simulink library "SUB_PLANT_Chassis"  (R2018a)
settings: Solver=VariableStepAuto  StartTime=0.0  StopTime=10.0  RelTol=1e-3
values from neighbouring files (symbols this model uses):
  Cf = 120000    [SUB_PLANT_LateralDynamics_CAL.mat]
  Cr = 240000    [SUB_PLANT_LateralDynamics_CAL.mat]
  GLB_FIXED_STEP_SIZE_CPV = ptc_matlab_lib.PTC_MBDS_Parameter('Value', 0.01,  	'Description', 'Global Fixed Step Size (Fundamental Sample Time)',  	'Unit', 's',  	'CoderInfo.StorageClass', 'Custom',  	'CoderInfo.CustomStorageClass', 'Const')    [GLB_CONST.m]
  heading_0 = 5.2    [SUB_PLANT_LateralDynamics_CAL.mat]
  Iz = 10000    [SUB_PLANT_LateralDynamics_CAL.mat]
  lf = 2.5    [SUB_PLANT_LateralDynamics_CAL.mat]
  lr = 3.5    [SUB_PLANT_LateralDynamics_CAL.mat]
  Vx_0 = 1    [SUB_PLANT_LateralDynamics_CAL.mat]
undefined symbols (not defined in the file or in its folder): DiscIntNeverNeededParam, GLB_TRANS_LOSS_TRQ_GEAR_STEP_MPV, GLB_TRANS_LOSS_TRQ_SPD_STEP_MPV, GLB_TRANS_LOSS_TRQ_TABLE_DATA_MPV, GLB_TRANS_LOSS_TRQ_TRQ_STEP_MPV
libraries: PTC_MBDS_LIB x41, simulink x6
(part 2 of 2)

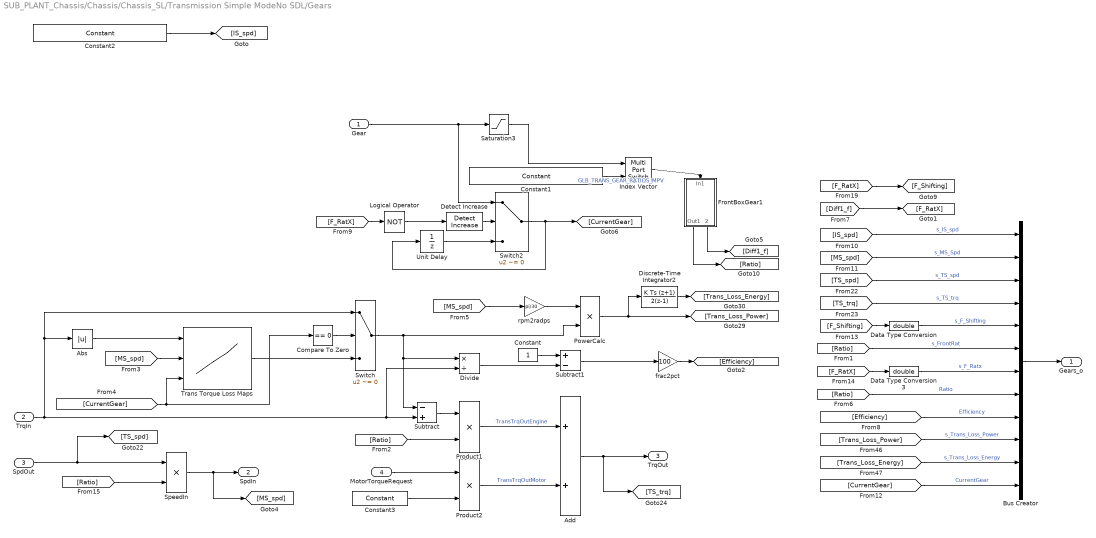
== system SUB_PLANT_Chassis/Chassis/Chassis_SL/Transmission Simple ModeNo SDL/Gears ==
  Gear : Inport
  TrqIn : Inport  Port=2
  SpdOut : Inport  Port=3
  MotorTorqueRequest : Inport  Port=4
  Abs : Abs
  Add : Sum
  Bus Creator : BusCreator  Inputs=12
  Compare To Zero : simulink/Logic and Bit Operations/Compare To Zero  relop===  OutDataTypeStr=boolean
  Constant : Constant
  Constant1 : PTC_MBDS_LIB/Extras/Sources/Constant  Value2=GLB_TRANS_GEAR_RATIOS_MPV  PTC_MBDS_BlockVersion=5.41  PTC_BlockType=PTC_MBDS_Constant
      settings: SourceProductName=PACCAR Technical Center MBDS Library
      settings: AttributesFormatString=|
      | Value: <1 X 12>
      | Unit: '1'
  Constant2 : PTC_MBDS_LIB/Extras/Sources/Constant  Value2=0  PTC_MBDS_BlockVersion=5.41  PTC_BlockType=PTC_MBDS_Constant
      settings: SourceProductName=PACCAR Technical Center MBDS Library
  Constant3 : PTC_MBDS_LIB/Extras/Sources/Constant  Value2=1  PTC_MBDS_BlockVersion=5.41  PTC_BlockType=PTC_MBDS_Constant
      settings: SourceProductName=PACCAR Technical Center MBDS Library
  Data Type Conversion : DataTypeConversion  OutDataTypeStr=double
  Data Type Conversion3 : DataTypeConversion  OutDataTypeStr=double
  Detect Increase : simulink/Logic and Bit Operations/Detect Increase  vinit=0.0  OutDataTypeStr=boolean
  Discrete-Time Integrator2 : DiscreteIntegrator  IntegratorMethod=Integration: Trapezoidal  SampleTime=GLB_FIXED_STEP_SIZE_CPV  ICPrevOutput=DiscIntNeverNeededParam  ICPrevScaledInput=DiscIntNeverNeededParam
  Divide : Product  Inputs=*/
  FrontBoxGear1 : Subsystem
  Index Vector : MultiPortSwitch  Inputs=1
  Logical Operator : Logic  Operator=NOT  AllPortsSameDT=off  OutDataTypeStr=boolean
  PowerCalc : Product
  Product1 : Product
  Product2 : Product
  Saturation3 : Saturate  UpperLimit=inf  LowerLimit=1
  SpeedIn : Product
  Subtract : Sum  Inputs=-+
  Subtract1 : Sum  Inputs=+-
  Switch : Switch  Criteria=u2 ~= 0
  Switch2 : Switch  Criteria=u2 ~= 0
  Trans Torque Loss Maps : Lookup_n-D  NumberOfTableDimensions=3  BreakpointsForDimension1=GLB_TRANS_LOSS_TRQ_TRQ_STEP_MPV  BreakpointsForDimension2=GLB_TRANS_LOSS_TRQ_SPD_STEP_MPV  BreakpointsForDimension3=GLB_TRANS_LOSS_TRQ_GEAR_STEP_MPV  BeginIndexSearchUsingPreviousIndexResult=on  Table=GLB_TRANS_LOSS_TRQ_TABLE_DATA_MPV  InternalRulePriority=Speed  RndMeth=Simplest  InputSameDT=on
  Unit Delay : UnitDelay  SampleTime=-1
  frac2pct : Gain  Gain=100
  rpm2radps : Gain  Gain=pi/30
  Gears_o : Outport
  SpdIn : Outport  Port=2
  TrqOut : Outport  Port=3
  wires:
  Constant3/1 -> Product2/2
  Product2/1 -> Add/2  "TransTrqOutMotor"
  Product1/1 -> Add/1  "TransTrqOutEngine"
  MotorTorqueRequest/1 -> Product2/1
  [Trans_Loss_Energy] -> Bus Creator/11  "s_Trans_Loss_Energy"
  [Trans_Loss_Power] -> Bus Creator/10  "s_Trans_Loss_Power"
  [Efficiency] -> Bus Creator/9  "Efficiency"
  Data Type Conversion3/1 -> Bus Creator/7  "s_F_Ratx"
  [Ratio] -> Bus Creator/6  "s_FrontRat"
  Data Type Conversion/1 -> Bus Creator/5  "s_F_Shifting"
  Constant1/1 -> Index Vector/2  "GLB_TRANS_GEAR_RATIOS_MPV"
  Discrete-Time Integrator2/1 -> [Trans_Loss_Energy]
  PowerCalc/1 -> [Trans_Loss_Power], Discrete-Time Integrator2/1
  [Diff1_f] -> [F_RatX]
  SpdOut/1 -> [TS_spd], SpeedIn/1
  FrontBoxGear1/2(Diff_F) -> [Diff1_f]
  FrontBoxGear1/1(Out1) -> [Ratio]
  [F_RatX] -> [F_Shifting]
  [F_RatX] -> Data Type Conversion3/1
  Gear/1 -> Switch2/1, Saturation3/1
  Index Vector/1 -> FrontBoxGear1/1(In1)
  [IS_spd] -> Bus Creator/1  "s_IS_spd"
  [MS_spd] -> Bus Creator/2  "s_MS_Spd"
  [TS_spd] -> Bus Creator/3  "s_TS_spd"
  [TS_trq] -> Bus Creator/4  "s_TS_trq"
  [F_Shifting] -> Data Type Conversion/1
  Bus Creator/1 -> Gears_o/1
  Unit Delay/1 -> Switch2/3
  Logical Operator/1 -> Detect Increase/1
  [F_RatX] -> Logical Operator/1
  Switch2/1 -> [CurrentGear], Unit Delay/1
  Detect Increase/1 -> Switch2/2
  [CurrentGear] -> Bus Creator/12  "CurrentGear"
  [Ratio] -> Product1/2
  [Ratio] -> SpeedIn/2
  SpeedIn/1 -> [MS_spd], SpdIn/1
  Add/1 -> TrqOut/1, [TS_trq]
  Saturation3/1 -> Index Vector/1
  [MS_spd] -> Trans Torque Loss Maps/2
  Switch/1 -> PowerCalc/2, Divide/1, Subtract/1
  [MS_spd] -> rpm2radps/1
  rpm2radps/1 -> PowerCalc/1
  Subtract1/1 -> frac2pct/1
  frac2pct/1 -> [Efficiency]
  [CurrentGear] -> Trans Torque Loss Maps/3, Compare To Zero/1
  Abs/1 -> Trans Torque Loss Maps/1
  Trans Torque Loss Maps/1 -> Switch/3
  Compare To Zero/1 -> Switch/2
  [Ratio] -> Bus Creator/8  "Ratio"
  TrqIn/1 -> Subtract/2, Divide/2, Switch/1, Abs/1
  Constant/1 -> Subtract1/1
  Divide/1 -> Subtract1/2
  Subtract/1 -> Product1/1
  Constant2/1 -> [IS_spd]

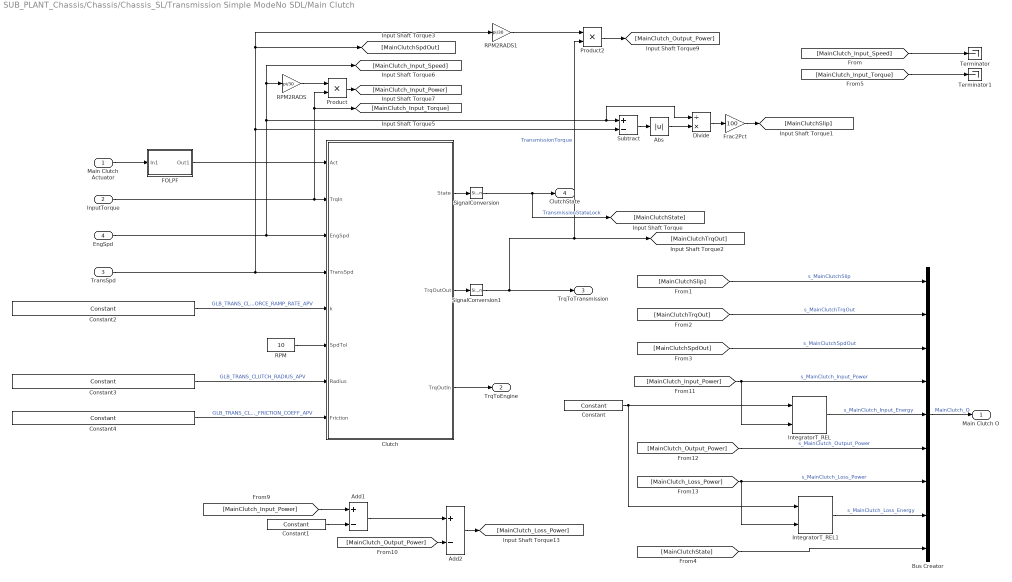
== system SUB_PLANT_Chassis/Chassis/Chassis_SL/Transmission Simple ModeNo SDL/Main Clutch ==
  Main Clutch Actuator : Inport
  InputTorque : Inport  Port=2
  TransSpd : Inport  Port=3
  EngSpd : Inport  Port=4
  Abs : Abs
  Add1 : Sum  Inputs=+-
  Add2 : Sum  Inputs=+-
  Bus Creator : BusCreator  Inputs=9
  Clutch : Stateflow chart  TreatAsAtomicUnit=on
  Constant : PTC_MBDS_LIB/Extras/Sources/Constant  Value2=1  PTC_MBDS_BlockVersion=5.41  PTC_BlockType=PTC_MBDS_Constant
      settings: SourceProductName=PACCAR Technical Center MBDS Library
  Constant1 : PTC_MBDS_LIB/Extras/Sources/Constant  Value2=0  PTC_MBDS_BlockVersion=5.41  PTC_BlockType=PTC_MBDS_Constant
      settings: SourceProductName=PACCAR Technical Center MBDS Library
  Constant2 : PTC_MBDS_LIB/Extras/Sources/Constant  Value2=GLB_TRANS_CLUTCH_FORCE_RAMP_RATE_APV  PTC_MBDS_BlockVersion=5.41  PTC_BlockType=PTC_MBDS_Constant
      settings: SourceProductName=PACCAR Technical Center MBDS Library
      settings: AttributesFormatString=|
      | Value: 5000
      | Unit: 'N/s'
  Constant3 : PTC_MBDS_LIB/Extras/Sources/Constant  Value2=GLB_TRANS_CLUTCH_RADIUS_APV  PTC_MBDS_BlockVersion=5.41  PTC_BlockType=PTC_MBDS_Constant
      settings: SourceProductName=PACCAR Technical Center MBDS Library
      settings: AttributesFormatString=|
      | Value: 0.215
      | Unit: 'm'
  Constant4 : PTC_MBDS_LIB/Extras/Sources/Constant  Value2=GLB_TRANS_CLUTCH_FRICTION_COEFF_APV  PTC_MBDS_BlockVersion=5.41  PTC_BlockType=PTC_MBDS_Constant
      settings: SourceProductName=PACCAR Technical Center MBDS Library
      settings: AttributesFormatString=|
      | Value: 0.3
      | Unit: '1'
  Divide : Product  Inputs=/*
  FOLPF : Subsystem
  Frac2Pct : Gain  Gain=100
  IntegratorT_REL : PTC_MBDS_LIB/MBDS Standard Library/Extended Operations/Integrators/IntegratorT_REL  MXMN_Enabled=off  MX=Inf  MN=-Inf  dT_Enabled=off  dT=GLB_FIXED_STEP_SIZE_CPV  E_Enabled=off  R_Enabled=off  IV_Enabled=off  IV=0  B_min_Enabled=off  B_max_Enabled=off  PTC_MBDS_BlockVersion=5.41  PTC_BlockType=PTC_MBDS_IntegratorT_REL
      settings: SourceProductName=PACCAR Technical Center MBDS Library
      settings: AttributesFormatString=|
      | IV = %<IV>
      | MN = %<MN>
      | MX = %<MX>
      | dT = %<dT>
  IntegratorT_REL1 : PTC_MBDS_LIB/MBDS Standard Library/Extended Operations/Integrators/IntegratorT_REL  MXMN_Enabled=off  MX=Inf  MN=-Inf  dT_Enabled=off  dT=GLB_FIXED_STEP_SIZE_CPV  E_Enabled=off  R_Enabled=off  IV_Enabled=off  IV=0  B_min_Enabled=off  B_max_Enabled=off  PTC_MBDS_BlockVersion=5.41  PTC_BlockType=PTC_MBDS_IntegratorT_REL
      settings: SourceProductName=PACCAR Technical Center MBDS Library
      settings: AttributesFormatString=|
      | IV = %<IV>
      | MN = %<MN>
      | MX = %<MX>
      | dT = %<dT>
  Product : Product  RndMeth=Zero
  Product2 : Product  RndMeth=Zero
  RPM : Constant  Value=10
  RPM2RADS : Gain  Gain=pi/30
  RPM2RADS1 : Gain  Gain=pi/30
  SignalConversion : SignalConversion  ConversionOutput=Contiguous copy  OverrideOpt=off
  SignalConversion1 : SignalConversion  ConversionOutput=Contiguous copy  OverrideOpt=off
  Subtract : Sum  Inputs=+-
  Terminator : Terminator
      settings: InitFcn=|
      | try
      |    MBDS_BlockCallback('Update', gcb);
      | end
  Terminator1 : Terminator
      settings: InitFcn=|
      | try
      |    MBDS_BlockCallback('Update', gcb);
      | end
  Main Clutch O : Outport
  TrqToEngine : Outport  Port=2
  TrqToTransmission : Outport  Port=3
  ClutchState : Outport  Port=4
  wires:
  IntegratorT_REL/1 -> Bus Creator/5  "s_MainClutch_Input_Energy"
  IntegratorT_REL1/1 -> Bus Creator/8  "s_MainClutch_Loss_Energy"
  [MainClutch_Loss_Power] -> IntegratorT_REL1/2, Bus Creator/7  "s_MainClutch_Loss_Power"
  [MainClutch_Output_Power] -> Bus Creator/6  "s_MainClutch_Output_Power"
  [MainClutch_Input_Power] -> IntegratorT_REL/2, Bus Creator/4  "s_MainClutch_Input_Power"
  Add2/1 -> [MainClutch_Loss_Power]
  Add1/1 -> Add2/1
  [MainClutch_Output_Power] -> Add2/2
  [MainClutch_Input_Power] -> Add1/1
  Product2/1 -> [MainClutch_Output_Power]
  Product/1 -> [MainClutch_Input_Power]
  Main Clutch Actuator/1 -> FOLPF/1(In1)
  Bus Creator/1 -> Main Clutch O/1  "MainClutch_O"
  [MainClutchSlip] -> Bus Creator/1  "s_MainClutchSlip"
  [MainClutchTrqOut] -> Bus Creator/2  "s_MainClutchTrqOut"
  [MainClutchSpdOut] -> Bus Creator/3  "s_MainClutchSpdOut"
  Frac2Pct/1 -> [MainClutchSlip]
  Clutch/3(TrqOutIn) -> TrqToEngine/1
  Clutch/2(TrqOutOut) -> SignalConversion1/1
  InputTorque/1 -> Clutch/2(TrqIn), Product/2, [MainClutch_Input_Torque]
  EngSpd/1 -> Clutch/3(EngSpd), Divide/1, Subtract/1, [MainClutch_Input_Speed], RPM2RADS/1
  RPM/1 -> Clutch/6(SpdTol)
  FOLPF/1(Out1) -> Clutch/1(Act)
  Clutch/1(State) -> SignalConversion/1
  RPM2RADS/1 -> Product/1
  RPM2RADS1/1 -> Product2/1
  Divide/1 -> Frac2Pct/1
  Abs/1 -> Divide/2
  Subtract/1 -> Abs/1
  TransSpd/1 -> Clutch/4(TransSpd), Subtract/2, RPM2RADS1/1, [MainClutchSpdOut]
  Constant4/1 -> Clutch/8(Friction)  "GLB_TRANS_CLUTCH_FRICTION_COEFF_APV"
  Constant3/1 -> Clutch/7(Radius)  "GLB_TRANS_CLUTCH_RADIUS_APV"
  Constant/1 -> IntegratorT_REL1/1, IntegratorT_REL/1
  Constant1/1 -> Add1/2
  [MainClutchState] -> Bus Creator/9
  [MainClutch_Input_Speed] -> Terminator/1
  [MainClutch_Input_Torque] -> Terminator1/1
  SignalConversion/1 -> ClutchState/1, [MainClutchState]  "TransmissionStateLock"
  SignalConversion1/1 -> Product2/2, [MainClutchTrqOut], TrqToTransmission/1  "TransmissionTorque"
  Constant2/1 -> Clutch/5(k)  "GLB_TRANS_CLUTCH_FORCE_RAMP_RATE_APV"

== system SUB_PLANT_Chassis/Chassis/Chassis_SL/Chassis/Vehicle Dynamics/Aero ==
  note: Density
      | of Air
  Rho : Inport
  Cd : Inport  Port=2
  Af : Inport  Port=3
  xDot : Inport  Port=4
  Gain3 : Gain  Gain=0.5
  Product : Product
  Product2 : Product
  Product3 : Product
  Signed square : Subsystem
      mask Display: fprintf('Signed\nsquare')
  AeroDragForce : Outport
  wires:
  xDot/1 -> Signed square/1(In1)
  Product3/1 -> AeroDragForce/1
  Gain3/1 -> Product/2
  Signed square/1(Out1) -> Gain3/1
  Rho/1 -> Product/1
  Product/1 -> Product2/2
  Cd/1 -> Product2/1
  Product2/1 -> Product3/2
  Af/1 -> Product3/1

== system SUB_PLANT_Chassis/Chassis/Chassis_SL/Transmission Simple ModeNo SDL/Gears/FrontBoxGear1 ==
  In1 : Inport
  Abs : Abs
  Constant : PTC_MBDS_LIB/Extras/Sources/Constant  Value2=0.2  PTC_MBDS_BlockVersion=5.41  PTC_BlockType=PTC_MBDS_Constant
      settings: SourceProductName=PACCAR Technical Center MBDS Library
  LowpassT_RE : PTC_MBDS_LIB/MBDS Standard Library/Extended Operations/Filters/LowpassT_RE  dT_Enabled=off  dT=GLB_FIXED_STEP_SIZE_CPV  E_Enabled=off  R_Enabled=off  IV_Enabled=off  IV=0  PTC_MBDS_BlockVersion=5.41  PTC_BlockType=PTC_MBDS_LowpassT_RE
      settings: SourceProductName=PACCAR Technical Center MBDS Library
      settings: AttributesFormatString=|
      | IV = %<IV>
      | dT = %<dT>
  Relational Operator : RelationalOperator  OutDataTypeStr=boolean  RndMeth=Nearest
  Saturation : Saturate  UpperLimit=inf  LowerLimit=.1
  Subtract : Sum  Inputs=-+
  TransMdlMaxRatDelta : Constant  Value=.01
  Out1 : Outport
  Diff_F : Outport  Port=2
  wires:
  Subtract/1 -> Abs/1
  Abs/1 -> Relational Operator/1
  TransMdlMaxRatDelta/1 -> Relational Operator/2
  Relational Operator/1 -> Diff_F/1
  Saturation/1 -> Out1/1
  LowpassT_RE/1 -> Subtract/1, Saturation/1
  In1/1 -> LowpassT_RE/2, Subtract/2
  Constant/1 -> LowpassT_RE/1

== system SUB_PLANT_Chassis/Chassis/Chassis_SL/Transmission Simple ModeNo SDL/Main Clutch/FOLPF ==
  In1 : Inport
  Add1 : Sum  Inputs=+-
  Add2 : Sum
  Constant : Constant  Value=.95
  Constant1 : Constant
  Product : Product
  Product1 : Product
  Unit Delay : UnitDelay  SampleTime=-1
  Out1 : Outport
  wires:
  Constant1/1 -> Add1/1
  Add1/1 -> Product/2
  Product/1 -> Add2/1
  In1/1 -> Product/1
  Product1/1 -> Add2/2
  Unit Delay/1 -> Product1/2
  Constant/1 -> Add1/2, Product1/1
  Add2/1 -> Out1/1, Unit Delay/1

== system SUB_PLANT_Chassis/Chassis/Chassis_SL/Chassis/Vehicle Dynamics/Aero/Signed square ==
  In1 : Inport
  Math Function : Math  Operator=square  SaturateOnIntegerOverflow=on
  Product : Product  RndMeth=Zero
  Sign : Signum  ZeroCross=off
  Out1 : Outport
  wires:
  In1/1 -> Math Function/1, Sign/1
  Math Function/1 -> Product/1
  Sign/1 -> Product/2
  Product/1 -> Out1/1

== matlab function SUB_PLANT_Chassis/Chassis/Chassis_SL/Chassis/Trailer Model/wrap to pi1 ==
  data: u input; y output
function y = fcn(u)
if (u>pi)
    y=u-2*pi;
elseif (u<-pi)
    y=u+2*pi;
else
    y=u;
end

== stateflow chart SUB_PLANT_Chassis/Chassis/Chassis_SL/Transmission Simple ModeNo SDL/Main Clutch/Clutch ==
  state Init
    entry: State=1;
  state Open
    entry: State=2;
    entry: ClutchForce=0;
    during:TrqOutOut=0;
    during:TrqOutIn=0;
  state ReverseSlip
    en:State=4;
    during:ClutchForce = ClutchForce + k*GLB_FIXED_STEP_SIZE_CPV;
    during:TrqOutIn=-2/3*Radius*Friction*ClutchForce;
    during:TrqOutOut=TrqOutOut;
  state ForwardSlip
    en:State=3;
    during:ClutchForce = ClutchForce + k*GLB_FIXED_STEP_SIZE_CPV;
    during:TrqOutOut=2/3*Radius*Friction*ClutchForce;
    during:TrqOutIn=TrqOutOut;
  state Locked
    en:State=5;
    entry: ClutchForce=10000;
    during:TrqOutOut=TrqIn;
    during:TrqOutIn=0;
  (default) -> Init
  Init -> Open
  ReverseSlip -> Open [order 1] : [Act<0.5]
  Locked -> Open : [Act<0.5]
  ForwardSlip -> Open [order 2] : [Act<0.5]
  Open -> (junction 29) : [Act>=0.5]
  (junction 29) -> ReverseSlip [order 2] : [EngSpd<TransSpd]
  (junction 29) -> ForwardSlip [order 1] : [EngSpd>=TransSpd]
  ReverseSlip -> ForwardSlip [order 3] : [EngSpd>=TransSpd]
  ForwardSlip -> ReverseSlip [order 3] : [EngSpd<TransSpd]
  ReverseSlip -> Locked [order 2] : [abs(EngSpd-TransSpd)<SpdTol]
  ForwardSlip -> Locked [order 1] : [abs(EngSpd-TransSpd)<SpdTol]
  data: Act input; State output; TrqIn input; EngSpd input; TransSpd input; TrqOutOut output; k input; SpdTol input; TrqOutIn output; Radius input size=1; Friction input size=1; ClutchForce local; GLB_FIXED_STEP_SIZE_CPV parameter
